simulink model "engine_model"  (R2024b)
settings: Solver=VariableStepAuto  StartTime=0.0  StopTime=t_sim  RelTol=1e-6
values from neighbouring files (symbols this model uses):
  t_sim = 10    [main.m]
  x0 = [pman0; n0; mffdot0; lambda0]    [linearization_analysis.m]    (also in main.m = [0.5 * params(7); 3000; 3e-5; 14])
undefined symbols (not defined in the file or in its folder): alpha_ref, lambda_ref, mfi_dot_ref, params
settings Model: Creator=giovanni.mattei  LastModifiedBy=Giulia
settings SolverCC: MaxConsecutiveMinStep=10
settings DataIOCC: SaveFormat=Array
settings RTWCC: GPUComputeCapability=3.5

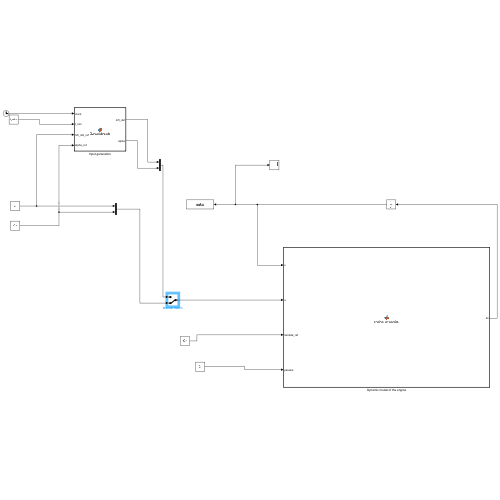
[thumbnail: Simulink's stored preview of the top-level diagram]
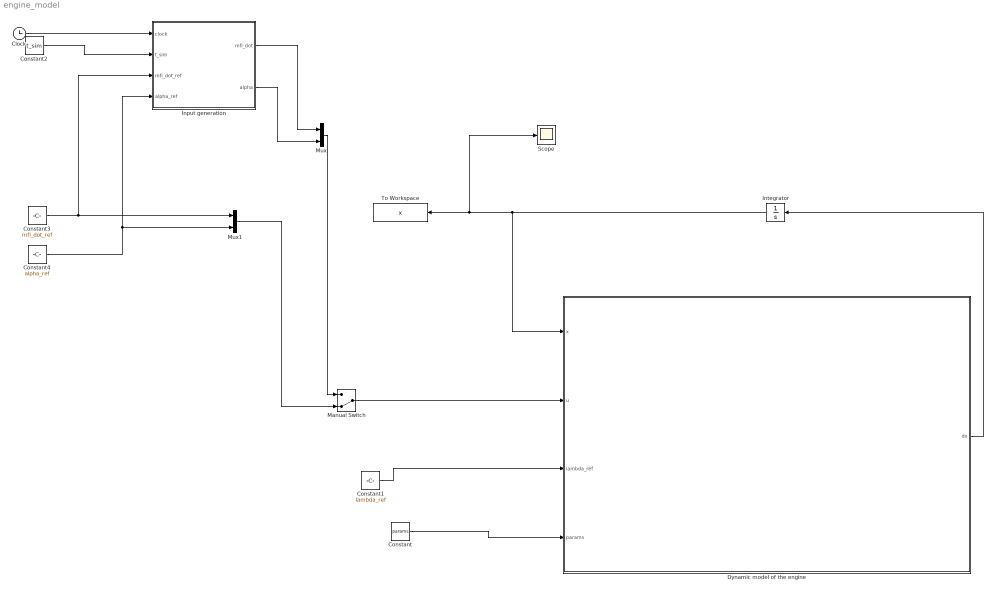
== system engine_model ==
  Clock : Clock
  Constant : Constant  Value=params
  Constant1 : Constant  Value=lambda_ref
  Constant2 : Constant  Value=t_sim
  Constant3 : Constant  Value=mfi_dot_ref
  Constant4 : Constant  Value=alpha_ref
  Dynamic model of the engine : MATLAB Function  TreatAsAtomicUnit=on
  Input generation : MATLAB Function  TreatAsAtomicUnit=on
  Integrator : Integrator  InitialCondition=x0
  Manual Switch : ManualSwitch  CurrentSetting=0
  Mux : Mux  Inputs=2
  Mux1 : Mux  Inputs=2
  Scope : Scope
  To Workspace : ToWorkspace  VariableName=x  SaveFormat=Timeseries  SampleTime=-1
  wires:
  Constant/1 -> Dynamic model of the engine/4(params)
  Dynamic model of the engine/1(dx) -> Integrator/1
  Integrator/1 -> Scope/1, To Workspace/1, Dynamic model of the engine/1(x)
  Clock/1 -> Input generation/1(clock)
  Constant1/1 -> Dynamic model of the engine/3(lambda_ref)
  Constant2/1 -> Input generation/2(t_sim)
  Constant3/1 -> Mux1/1, Input generation/3(mfi_dot_ref)
  Constant4/1 -> Mux1/2, Input generation/4(alpha_ref)
  Input generation/1(mfi_dot) -> Mux/1
  Input generation/2(alpha) -> Mux/2
  Manual Switch/1 -> Dynamic model of the engine/2(u)
  Mux/1 -> Manual Switch/1
  Mux1/1 -> Manual Switch/2

== matlab function engine_model/Input generation ==
  data: mfi_dot output; alpha output; clock input; t_sim input; mfi_dot_ref input; alpha_ref input
function [mfi_dot, alpha] = DynamicInputs(clock, t_sim, mfi_dot_ref, alpha_ref)
% DynamicInputs generates time-varying inputs alpha (throttle angle)
% and mfi_dot (fuel injection mass flow rate) based on the simulation clock.
%
% Inputs:
% - clock: Simulation time (in seconds)
%
% Outputs:
% - alpha: Throttle angle (in degrees)
% - mfi_dot: Fuel injection mass flow rate (in kg/s)

    % Define step and ramp behavior
    if clock <= t_sim/3
        % Phase 1: Initial conditions
        alpha = alpha_ref; % Constant throttle angle (degrees)
        mfi_dot = mfi_dot_ref; % Initial fuel injection mass flow rate (kg/s)
    else
        % Phase 2: Acceleration (after 3 seconds)
        alpha = alpha_ref + 5 * (clock - t_sim/3); % Ramp throttle angle (degrees)
        mfi_dot = 3*mfi_dot_ref; % Increased fuel injection (kg/s)
    end
end

== matlab function engine_model/Dynamic model of the engine ==
  data: x input; u input; lambda_ref input; params input; dx output
function dx = engine_dynamics(x, u, lambda_ref, params)
    % Engine dynamics 
    %
    % Inputs:
    %   x - State vector [p; n; m_ff; lambda_m]
    %       n: Engine (crank shaft) speed (rpm)
    %       m_ff: Fuel-film mass flow-rate (Kg)
    %       lambda_m: measured air-fuel ratio
    %       p: Intake manifold pressure (Pa)
    %   u - Control input vector [mf_dot; alpha]
    %       mf_dot: Injected fuel mass flow (Kg/s)
    %       alpha: Throttle plate angle (degrees)
    %   params - Vector of engine parameters
    %
    % Output:
    %   dx - Derivative of the state vector

    % Extract states
    p_man = x(1);
    n = x(2);
    m_ff = x(3);
    lambda_m = x(4);
    
    % Extract inputs
    mfi_dot = u(1);
    alpha = deg2rad(u(2)); % Convert angle to radians

    % Extract parameters
    T_man = params(1);
    V = params(2);
    V_d = params(3);
    R = params(4);
    C_t = params(5);
    D = params(6);
    p_amb = params(7);
    T_amb = params(8);
    alpha0 = deg2rad(params(9));
    k = params(10);
    eta_vn0 = params(11);
    eta_vn1 = params(12);
    eta_vn2 = params(13);
    eta_vp1 = params(14);
    %lambda_s = params(15);
    N = params(16);
    a = params(17);
    Hu = params(18); 
    eta_b = params(19);
    I = params(20);
    C = params(21);
    Pb = params(22);

    % Fuel film dynamics parameters
    sigma3 = 1.67;       % Parametro \sigma_3
    sigma4 = 0.65;       % Parametro \sigma_4
    sigma5 = 9.6e-5;     % Parametro \sigma_5
    sigma6 = 0.7236;     % Parametro \sigma_6

    % tau_f and chi based on reference engine speed
    tau_f = sigma3 * n^(-sigma4); % Costante di tempo del film di carburante
    chi = sigma5 * n + sigma6;    % Frazione del carburante vaporizzato

    % Calculate beta1(alpha) 
    beta1_alpha = (1 - cos(alpha) / cos(alpha0)) + ...
                  (2 / pi) * ((a / cos(alpha)) * ...
                  sqrt(cos(alpha)^2 - a^2 * cos(alpha0)^2)) + ...
                  (2 / pi) * (((cos(alpha) / cos(alpha0)) * ...
                  asin(a * cos(alpha0) / cos(alpha)) - a * sqrt(1 - a^2) - asin(a)));

    % Calculate beta2(p/p_amb) 
    p_crit = p_man / p_amb;
    if p_crit >= (2 / (k + 1))^(k / (k - 1))
        beta2_p = sqrt((2 * k / (k - 1)) * (p_crit^(2 / k) - p_crit^((k + 1) / k)));
    else
        beta2_p = sqrt(k) * (2 / (k + 1))^((k + 1) / (2 * (k - 1)));
    end

    % Calculate volumetric efficiency eta_v 
    eta_v = eta_vn0 + eta_vn1 * n + eta_vn2 * n^2 + eta_vp1 * p_man;

    % Intake manifold air mass flow 
    mdot_air = (C_t * (pi / 4) * D^2 * p_amb / sqrt(R * T_amb)) * ...
               beta1_alpha * beta2_p;

    % Intake manifold pressure dynamics 
    dp_man_dt = -(n * V_d * eta_v * p_man / (120 * V)) + ...
             (R * T_man * mdot_air / V);

    % Crank shaft speed dynamics
    dn_dt = - Pb/(n*I) + (Hu * eta_b/(n*I))*mfi_dot;
    
    % Fuel film dynamics
    dm_ff = (1 / tau_f) * (-m_ff + chi * mfi_dot);

    % Lambda misurato
    %lambda_m =

    % Lambda dynamics 
    dlambda_m_dt = -C*lambda_m + C*lambda_ref;

    % Construct state derivative
    dx = [dp_man_dt; dn_dt; dm_ff; dlambda_m_dt];
end
